simulink model "TP4_Haldane"  (R2024b)
settings: Solver=VariableStepAuto  StartTime=0.0  StopTime=10.0  FixedStep=0.  RelTol=1e-3
values from neighbouring files (symbols this model uses):
  D = 0.1    [Main_entregable.m]
  states0 = [x0;s0]*1.5    [DatosModeloTP4.m]    (also in Main_entregable.m = [x0;s0;0;0]*1.5)
  v0 = 1    [DatosModeloTP4.m]
settings Model: Creator=tomii  LastModifiedBy=tomii

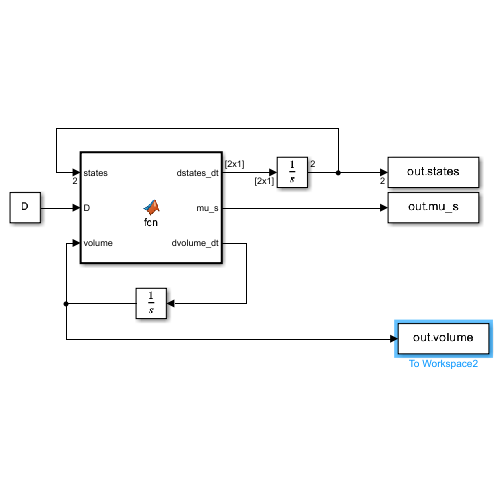
[thumbnail: Simulink's stored preview of the top-level diagram]
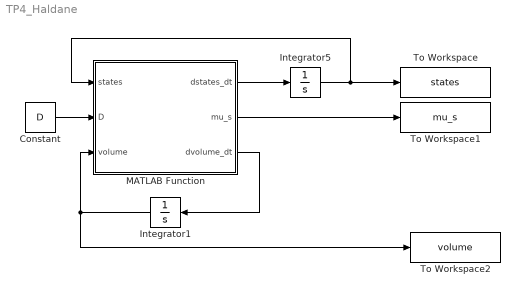
== system TP4_Haldane ==
  Constant : Constant  Value=D
  Integrator1 : Integrator  InitialCondition=v0
  Integrator5 : Integrator  InitialCondition=states0
  MATLAB Function : MATLAB Function  TreatAsAtomicUnit=on
  To Workspace : ToWorkspace  VariableName=states  SaveFormat=Timeseries  SampleTime=-1
  To Workspace1 : ToWorkspace  VariableName=mu_s  SaveFormat=Timeseries  SampleTime=-1
  To Workspace2 : ToWorkspace  VariableName=volume  SaveFormat=Timeseries  SampleTime=-1
  wires:
  MATLAB Function/1(dstates_dt) -> Integrator5/1
  Integrator5/1 -> MATLAB Function/1(states), To Workspace/1
  MATLAB Function/2(mu_s) -> To Workspace1/1
  Constant/1 -> MATLAB Function/2(D)
  MATLAB Function/3(dvolume_dt) -> Integrator1/1
  Integrator1/1 -> MATLAB Function/3(volume), To Workspace2/1

== matlab function TP4_Haldane/MATLAB Function ==
  data: dstates_dt output; mu_s output; states input; D input; volume input; modelParameters parameter; dvolume_dt output
function [dstates_dt, mu_s, dvolume_dt] = fcn(states, D, volume, modelParameters)   
    
    K=modelParameters.K;
    xi_in=modelParameters.xi_in;

    Ks=modelParameters.mu_model.Ks;
    Kis=modelParameters.mu_model.Kis;
    mu_max=modelParameters.mu_model.mu_max;
    
    x=states(1);
    s=states(2);

    mu_s=mu_max*(s/(s+Ks+s*s/Kis));
    rx=x*mu_s;

    dstates_dt = K * rx + D*(xi_in-states);
    dvolume_dt = volume*D;

end
